simulink model "Week1_Q5"  (R2020b)
settings: Solver=VariableStepAuto  StartTime=0.0  StopTime=10.0  RelTol=1e-3
values from neighbouring files (symbols this model uses):
  C = 10*10^-6    (= 1e-05)    [Variables.m]
  R = 20    [Variables.m]
settings Model: Creator=vikas  LastModifiedBy=vikas

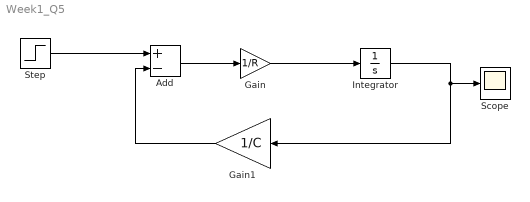
== system Week1_Q5 ==
  Add : Sum  Inputs=+-
  Gain : Gain  Gain=1/R
  Gain1 : Gain  Gain=1/C
  Integrator : Integrator  InitialCondition=8
  Scope : Scope
  Step : Step  SampleTime=0
  wires:
  Gain1/1 -> Add/2
  Gain/1 -> Integrator/1
  Add/1 -> Gain/1
  Integrator/1 -> Gain1/1, Scope/1
  Step/1 -> Add/1
